simulink model "trabControle17a"  (R2017a)
settings: Solver=VariableStepAuto  StartTime=0.0  StopTime=150  RelTol=1e-3
settings Model: Creator=iagof  LastModifiedBy=iagof
settings SFSimCC: SimUseLocalCustomCode=on
settings RTWCC: RTWUseLocalCustomCode=on

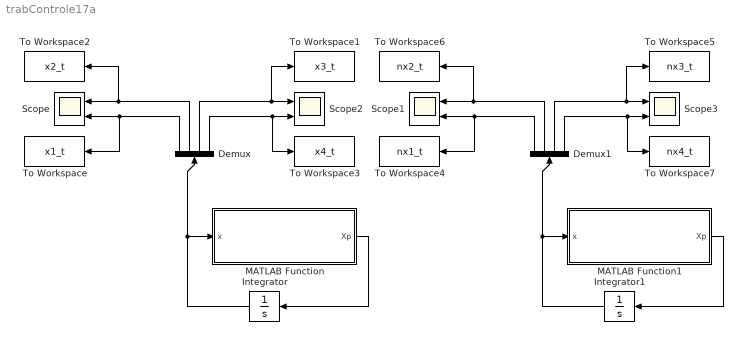
== system trabControle17a ==
  Demux : Demux
  Demux1 : Demux
  Integrator : Integrator  InitialCondition=[pi/3 0 0.1 0]
  Integrator1 : Integrator  InitialCondition=[pi/3 0 0.1 0]
  MATLAB Function : MATLAB Function  TreatAsAtomicUnit=on
  MATLAB Function1 : MATLAB Function  TreatAsAtomicUnit=on
  Scope{,1..3} (4 alike) : Scope  NumInputPorts=2
  To Workspace : ToWorkspace  VariableName=x1_t  SampleTime=-1
  To Workspace1 : ToWorkspace  VariableName=x3_t  SampleTime=-1
  To Workspace2 : ToWorkspace  VariableName=x2_t  SampleTime=-1
  To Workspace3 : ToWorkspace  VariableName=x4_t  SampleTime=-1
  To Workspace4 : ToWorkspace  VariableName=nx1_t  SampleTime=-1
  To Workspace5 : ToWorkspace  VariableName=nx3_t  SampleTime=-1
  To Workspace6 : ToWorkspace  VariableName=nx2_t  SampleTime=-1
  To Workspace7 : ToWorkspace  VariableName=nx4_t  SampleTime=-1
  wires:
  MATLAB Function/1(Xp) -> Integrator/1
  Integrator/1 -> MATLAB Function/1(x), Demux/1
  Demux/1 -> To Workspace/1, Scope/2
  Demux/2 -> To Workspace2/1, Scope/1
  Demux/3 -> To Workspace1/1, Scope2/1
  Demux/4 -> To Workspace3/1, Scope2/2
  Integrator1/1 -> MATLAB Function1/1(x), Demux1/1
  MATLAB Function1/1(Xp) -> Integrator1/1
  Demux1/3 -> To Workspace5/1, Scope3/1
  Demux1/4 -> To Workspace7/1, Scope3/2
  Demux1/2 -> To Workspace6/1, Scope1/1
  Demux1/1 -> To Workspace4/1, Scope1/2

== matlab function trabControle17a/MATLAB Function1 ==
  data: x input; Xp output
function Xp = dinamicaSistemaComControle(x)
    
    A = [ 0, 1, 0, 0;
        -209/16, -225/8,   365/28, -475/8;
        0, 0, 0, 1;
        209/160,  45/16, -247/168,  95/16];    
    
Xp = A*x;

== matlab function trabControle17a/MATLAB Function ==
  data: x input; Xp output
function Xp = dinamicaSistemaSemControle(x)
    
    A = [ 0, 1, 0, 0;
        -21/4, 0, 5/56, 0;
        0, 0, 0, 1;
        21/40, 0, -59/336, 0];    
    
Xp = A*x;
